simulink model "Piper_sol"  (R2023b)
settings: Solver=ode3  StartTime=0.0  StopTime=1000  FixedStep=0.01  RelTol=1e-3
values from neighbouring files (symbols this model uses):
  Kd = 1    [Piper_par_sol.m]
  Ki = 0.005    [Piper_par_sol.m]
  Kp = 0.5    [Piper_par_sol.m]
undefined symbols (not defined in the file or in its folder): denP, numP
settings Model: Creator=jerome  LastModifiedBy=jerome
settings ModelReferenceCC: EnableRefExpFcnMdlSchedulingChecks=on

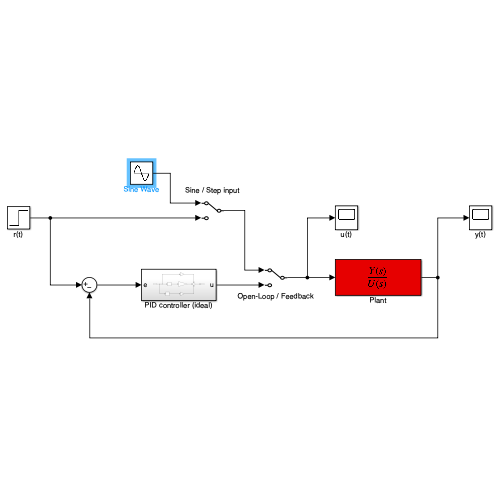
[thumbnail: Simulink's stored preview of the top-level diagram]
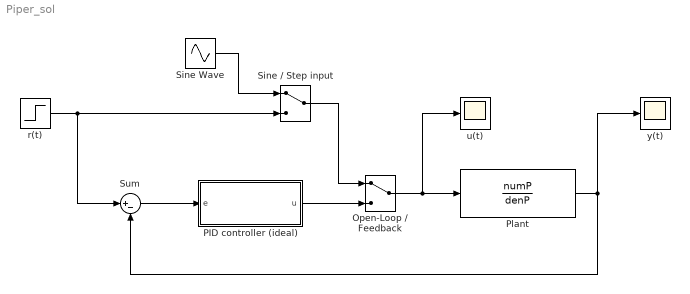
== system Piper_sol ==
  Open-Loop / Feedback : ManualSwitch
  PID controller (ideal) : Subsystem
  Plant : TransferFcn  Numerator=numP  Denominator=denP
  Sine / Step input : ManualSwitch
  Sine Wave : Sin  Frequency=0.241  SampleTime=0
  Sum : Sum  Inputs=|+-
  r(t) : Step  Time=0  SampleTime=0
  u(t) : Scope
  y(t) : Scope
  wires:
  Plant/1 -> Sum/2, y(t)/1
  Open-Loop / Feedback/1 -> u(t)/1, Plant/1
  r(t)/1 -> Sine / Step input/2, Sum/1
  PID controller (ideal)/1(u) -> Open-Loop / Feedback/2
  Sum/1 -> PID controller (ideal)/1(e)
  Sine / Step input/1 -> Open-Loop / Feedback/1
  Sine Wave/1 -> Sine / Step input/1

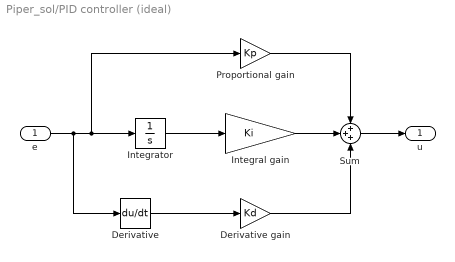
== system Piper_sol/PID controller (ideal) ==
  e : Inport
  Derivative : Derivative
  Derivative gain : Gain  Gain=Kd
  Integral gain : Gain  Gain=Ki
  Integrator : Integrator
  Proportional gain : Gain  Gain=Kp
  Sum : Sum  Inputs=+++
  u : Outport
  wires:
  Sum/1 -> u/1
  Proportional gain/1 -> Sum/1
  Derivative gain/1 -> Sum/3
  Integral gain/1 -> Sum/2
  e/1 -> Derivative/1, Proportional gain/1, Integrator/1
  Integrator/1 -> Integral gain/1
  Derivative/1 -> Derivative gain/1
